simulink model "Priklad_1"  (R2022b)
settings: Solver=VariableStepAuto  StartTime=0.0  StopTime=1000  RelTol=1e-3
settings Model: Creator=honza  LastModifiedBy=honza

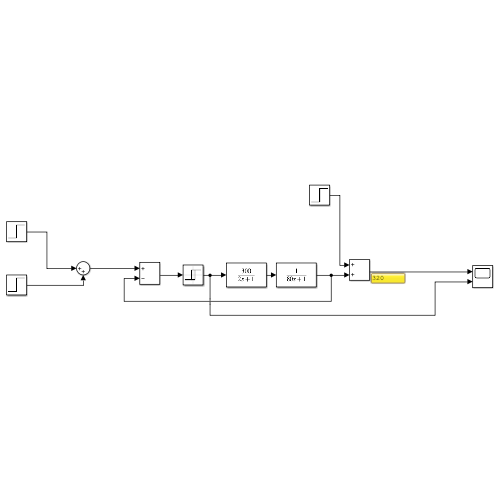
[thumbnail: Simulink's stored preview of the top-level diagram]
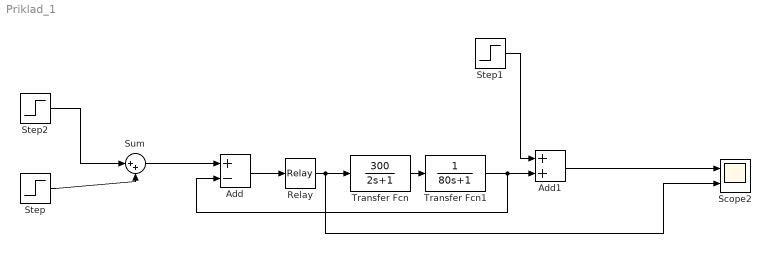
== system Priklad_1 ==
  Add : Sum  Inputs=+-
  Add1 : Sum
  Relay : Relay  OnSwitchValue=2  OffSwitchValue=-2
  Scope2 : Scope  NumInputPorts=2
  Step : Step  Time=0  After=180  SampleTime=0
  Step1 : Step  Time=0  After=20  SampleTime=0
  Step2 : Step  Time=300  After=250  SampleTime=0
  Sum : Sum  Inputs=|++
  Transfer Fcn : TransferFcn  Numerator=[300]  Denominator=[2 1]
  Transfer Fcn1 : TransferFcn  Denominator=[80 1]
  wires:
  Transfer Fcn/1 -> Transfer Fcn1/1
  Relay/1 -> Scope2/2, Transfer Fcn/1
  Add/1 -> Relay/1
  Transfer Fcn1/1 -> Add/2, Add1/2
  Add1/1 -> Scope2/1
  Sum/1 -> Add/1
  Step/1 -> Sum/2
  Step2/1 -> Sum/1
  Step1/1 -> Add1/1
